simulink model "SerieRuidoEntrada3"  (Simulink 7.2)
settings: Solver=ode3  StartTime=Intime  StopTime=Sttime  FixedStep=stime  RelTol=1e-3
values from neighbouring files (symbols this model uses):
  FTf = 1/mag*FTfp    [Filtros.m]    (also in RuidoFiltroN.m)
  FTf2 = 1/mag2*FTfp2    [Filtros.m]    (also in RuidoFiltroN.m)
  FTf3 = 1/mag3*FTfp3    [Filtros.m]
  FTf4 = 1/mag4*FTfp4    [Filtros.m]
  Intime = 0    [Filtros.m]    (also in RuidoFiltroN.m)
  stime = 10^-3    (= 0.001)    [Filtros.m]
  t2 = 15    [Filtros.m]
  t3 = 30    [Filtros.m]
  t4 = 35    [Filtros.m]
  tsub = 2    [Filtros.m]    (also in RuidoFiltroN.m)
libraries: simulink x1
settings Model: Creator=Ferdinando  LastModifiedBy=FVOliveira
settings DebuggingCC: StrictBusMsg=ErrorLevel1

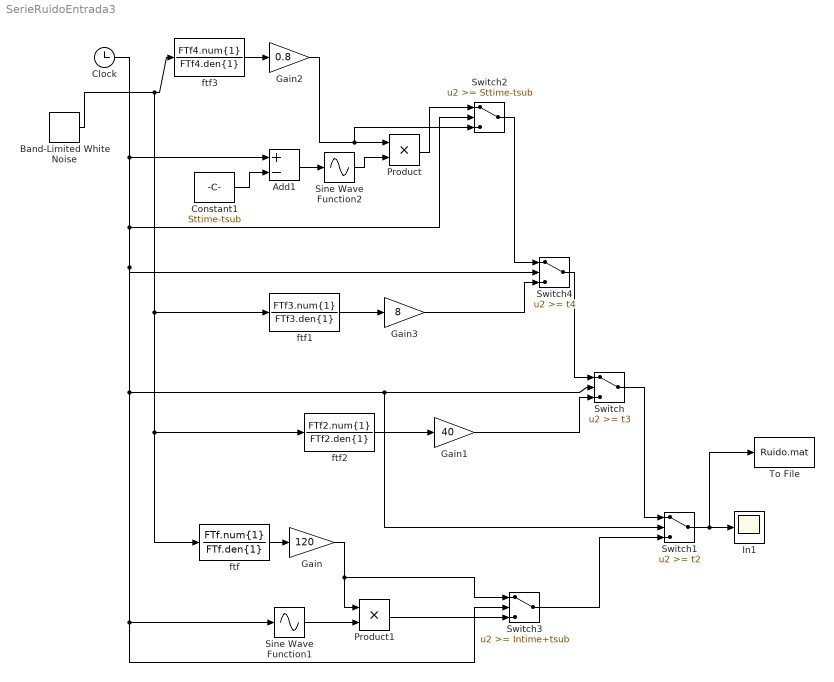
== system SerieRuidoEntrada3 ==
  Add1 : Sum  Inputs=+-  OutDataType=sfix(16)  OutScaling=2^-10
  Band-Limited White Noise : simulink/Sources/Band-Limited White Noise  SystemSampleTime=-1  Cov=[3.163*10^-5]  Ts=stime  seed=[23341]
  Clock : Clock
      settings: Decimation=10
  Constant1 : Constant  Value=Sttime-tsub  OutDataType=sfix(16)  OutScaling=2^0
  Gain : Gain  Gain=120  ParameterDataType=fixdt(1, 16)  ParameterScaling=2^0  OutDataType=fixdt(1, 16)  OutScaling=2^0
  Gain1 : Gain  Gain=40  ParameterDataType=fixdt(1, 16)  ParameterScaling=2^0  OutDataType=fixdt(1, 16)  OutScaling=2^0
  Gain2 : Gain  Gain=0.8  ParameterDataType=fixdt(1, 16)  ParameterScaling=2^0  OutDataType=fixdt(1, 16)  OutScaling=2^0
  Gain3 : Gain  Gain=8  ParameterDataType=fixdt(1, 16)  ParameterScaling=2^0  OutDataType=fixdt(1, 16)  OutScaling=2^0
  In1 : Scope
      settings: SaveName=Rand3and
  Product : Product  OutDataType=sfix(16)  OutScaling=2^0  RndMeth=Zero
  Product1 : Product  OutDataType=sfix(16)  OutScaling=2^0  RndMeth=Zero
  Sine Wave Function1 : Sin  TimeSource=Use external signal  Amplitude=0.5  Bias=0.5  Frequency=pi/tsub  Phase=-pi/2  SampleTime=0
  Sine Wave Function2 : Sin  TimeSource=Use external signal  Amplitude=0.5  Bias=0.5  Frequency=pi/tsub  Phase=pi/2  SampleTime=0
  Switch : Switch  Threshold=t3  OutDataType=fixdt(1, 16)  OutScaling=2^0
  Switch1 : Switch  Threshold=t2  OutDataType=fixdt(1, 16)  OutScaling=2^0
  Switch2 : Switch  Threshold=Sttime-tsub  OutDataType=fixdt(1, 16)  OutScaling=2^0
  Switch3 : Switch  Threshold=Intime+tsub  OutDataType=fixdt(1, 16)  OutScaling=2^0
  Switch4 : Switch  Threshold=t4  OutDataType=fixdt(1, 16)  OutScaling=2^0
  To File : ToFile  Filename=Ruido.mat  MatrixName=Ruido
  ftf : TransferFcn  Numerator=FTf.num{1}  Denominator=FTf.den{1}
  ftf1 : TransferFcn  Numerator=FTf3.num{1}  Denominator=FTf3.den{1}
  ftf2 : TransferFcn  Numerator=FTf2.num{1}  Denominator=FTf2.den{1}
  ftf3 : TransferFcn  Numerator=FTf4.num{1}  Denominator=FTf4.den{1}
  wires:
  Band-Limited White Noise/1 -> ftf2/1, ftf/1, ftf1/1, ftf3/1
  Clock/1 -> Add1/1, Switch2/2, Switch/2, Switch1/2, Switch3/2, Sine Wave Function1/1, Switch4/2
  ftf2/1 -> Gain1/1
  Switch/1 -> Switch1/1
  Switch1/1 -> In1/1, To File/1
  Sine Wave Function2/1 -> Product/2
  ftf3/1 -> Gain2/1
  Product/1 -> Switch2/1
  Switch3/1 -> Switch1/3
  Sine Wave Function1/1 -> Product1/2
  ftf/1 -> Gain/1
  Add1/1 -> Sine Wave Function2/1
  Constant1/1 -> Add1/2
  Product1/1 -> Switch3/3
  ftf1/1 -> Gain3/1
  Switch2/1 -> Switch4/1
  Switch4/1 -> Switch/1
  Gain2/1 -> Product/1, Switch2/3
  Gain3/1 -> Switch4/3
  Gain1/1 -> Switch/3
  Gain/1 -> Product1/1, Switch3/1
